simulink model "SH09"  (R2017b)
settings: Solver=VariableStepAuto  StartTime=0.0  StopTime=10.0  RelTol=1e-3
values from neighbouring files (symbols this model uses):
  SH09lin = FsClass.loadSH09_lin(dirWork, loadInitial)    [main.m]
settings Model: Creator=alejandro  LastModifiedBy=alejandro

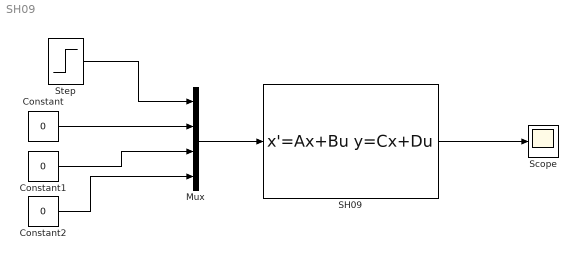
== system SH09 ==
  Constant : Constant  Value=0
  Constant1 : Constant  Value=0
  Constant2 : Constant  Value=0
  Mux : Mux
  SH09 : StateSpace  A=SH09lin.A  B=SH09lin.B  C=SH09lin.C  D=SH09lin.D  InitialCondition=0
  Scope : Scope
  Step : Step  SampleTime=0
  wires:
  Step/1 -> Mux/1
  Mux/1 -> SH09/1
  Constant/1 -> Mux/2
  Constant1/1 -> Mux/3
  Constant2/1 -> Mux/4
  SH09/1 -> Scope/1
